simulink model "FOG_v3_1"  (R2023b)
settings: Solver=ode4  StartTime=0.0  StopTime=0.02  FixedStep=2e-08  RelTol=1e-3
undefined symbols (not defined in the file): a_lp, b_lp, eta_conn, eta_dep, eta_K1, eta_pol, f_mod, K1_detector_ratio, K1_launch_ratio, K_norm, K_phase_to_deg, K_ref, K_sag, K_sagnac_power, Omega_deg_s, P_source_W, phi0, Rpd, Rtia, tau, visibility
settings Model: Creator=molik  LastModifiedBy=molik

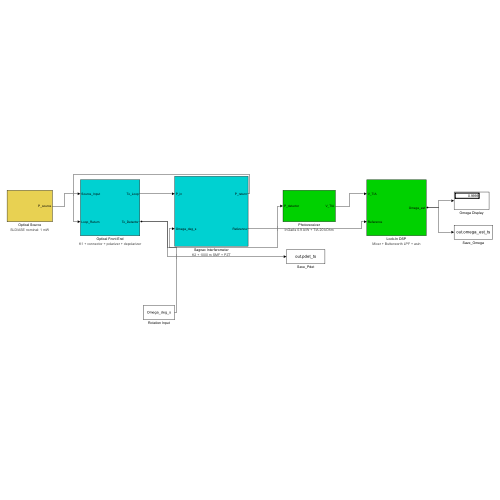
[thumbnail: Simulink's stored preview of the top-level diagram]
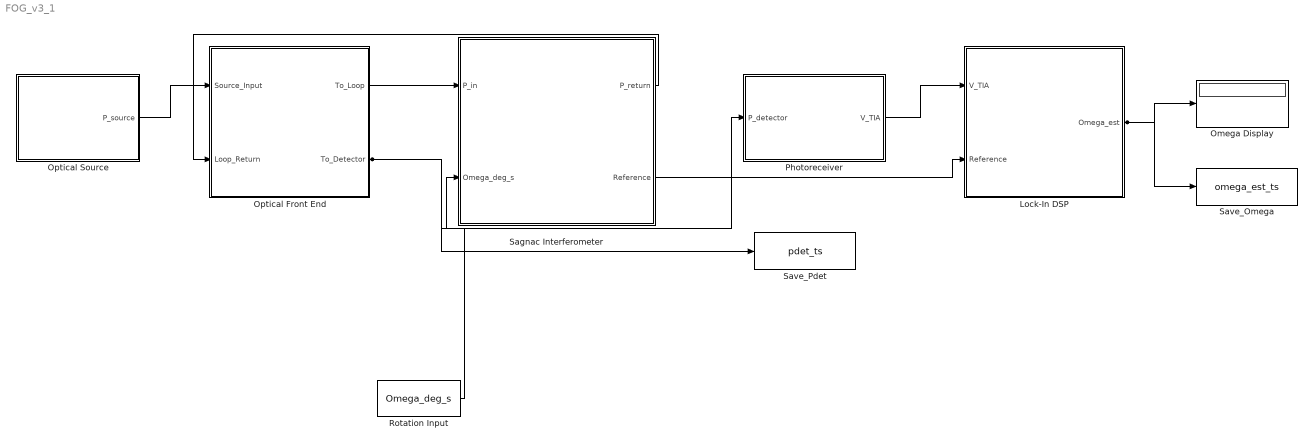
== system FOG_v3_1 ==
  Lock-In DSP : Subsystem
      settings: AttributesFormatString=Mixer + Butterworth LPF + asin
  Omega Display : Display
  Optical Front End : Subsystem
      settings: AttributesFormatString=K1 + connector + polarizer + depolarizer
  Optical Source : Subsystem
      settings: AttributesFormatString=SLD/ASE nominal: 1 mW
  Photoreceiver : Subsystem
      settings: AttributesFormatString=InGaAs 0.9 A/W + TIA 20 kOhm
  Rotation Input : Constant  Value=Omega_deg_s
  Sagnac Interferometer : Subsystem
      settings: AttributesFormatString=K2 + 1000 m SMF + PZT
  Save_Omega : ToWorkspace  VariableName=omega_est_ts  SaveFormat=Timeseries  SampleTime=-1
  Save_Pdet : ToWorkspace  VariableName=pdet_ts  SaveFormat=Timeseries  SampleTime=-1
  wires:
  Optical Source/1(P_source) -> Optical Front End/1(Source_Input)
  Optical Front End/1(To_Loop) -> Sagnac Interferometer/1(P_in)
  Rotation Input/1 -> Sagnac Interferometer/2(Omega_deg_s)
  Sagnac Interferometer/1(P_return) -> Optical Front End/2(Loop_Return)
  Optical Front End/2(To_Detector) -> Photoreceiver/1(P_detector), Save_Pdet/1
  Photoreceiver/1(V_TIA) -> Lock-In DSP/1(V_TIA)
  Sagnac Interferometer/2(Reference) -> Lock-In DSP/2(Reference)
  Lock-In DSP/1(Omega_est) -> Omega Display/1, Save_Omega/1

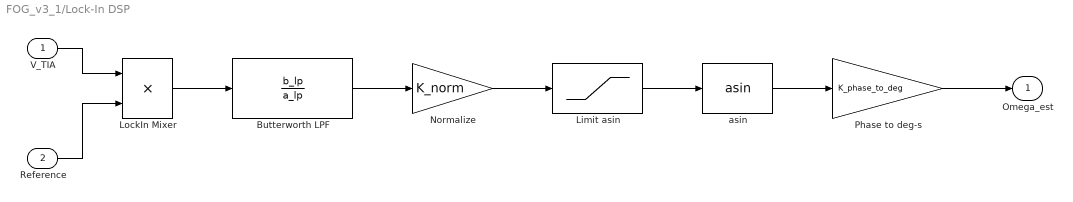
== system FOG_v3_1/Lock-In DSP ==
  V_TIA : Inport
  Reference : Inport  Port=2
  Butterworth LPF : TransferFcn  Numerator=b_lp  Denominator=a_lp
  Limit asin : Saturate  UpperLimit=0.999999  LowerLimit=-0.999999
  LockIn Mixer : Product
  Normalize : Gain  Gain=K_norm
  Phase to deg-s : Gain  Gain=K_phase_to_deg
  asin : Trigonometry  Operator=asin
  Omega_est : Outport
  wires:
  V_TIA/1 -> LockIn Mixer/1
  Reference/1 -> LockIn Mixer/2
  LockIn Mixer/1 -> Butterworth LPF/1
  Butterworth LPF/1 -> Normalize/1
  Normalize/1 -> Limit asin/1
  Limit asin/1 -> asin/1
  asin/1 -> Phase to deg-s/1
  Phase to deg-s/1 -> Omega_est/1

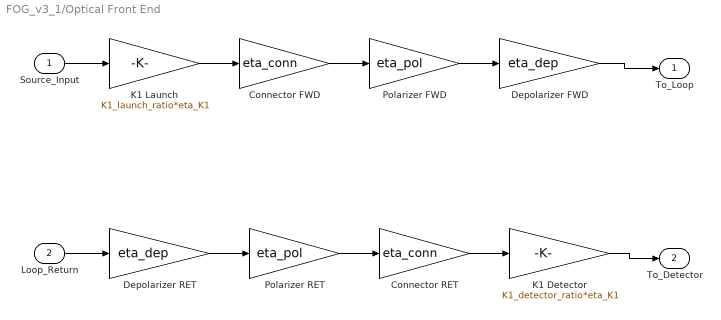
== system FOG_v3_1/Optical Front End ==
  Source_Input : Inport
  Loop_Return : Inport  Port=2
  Connector FWD : Gain  Gain=eta_conn
  Connector RET : Gain  Gain=eta_conn
  Depolarizer FWD : Gain  Gain=eta_dep
  Depolarizer RET : Gain  Gain=eta_dep
  K1 Detector : Gain  Gain=K1_detector_ratio*eta_K1
  K1 Launch : Gain  Gain=K1_launch_ratio*eta_K1
  Polarizer FWD : Gain  Gain=eta_pol
  Polarizer RET : Gain  Gain=eta_pol
  To_Loop : Outport
  To_Detector : Outport  Port=2
  wires:
  Source_Input/1 -> K1 Launch/1
  K1 Launch/1 -> Connector FWD/1
  Connector FWD/1 -> Polarizer FWD/1
  Polarizer FWD/1 -> Depolarizer FWD/1
  Depolarizer FWD/1 -> To_Loop/1
  Loop_Return/1 -> Depolarizer RET/1
  Depolarizer RET/1 -> Polarizer RET/1
  Polarizer RET/1 -> Connector RET/1
  Connector RET/1 -> K1 Detector/1
  K1 Detector/1 -> To_Detector/1

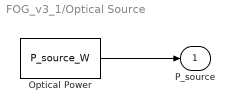
== system FOG_v3_1/Optical Source ==
  Optical Power : Constant  Value=P_source_W
  P_source : Outport
  wires:
  Optical Power/1 -> P_source/1

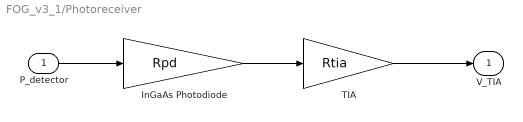
== system FOG_v3_1/Photoreceiver ==
  P_detector : Inport
  InGaAs Photodiode : Gain  Gain=Rpd
  TIA : Gain  Gain=Rtia
  V_TIA : Outport
  wires:
  P_detector/1 -> InGaAs Photodiode/1
  InGaAs Photodiode/1 -> TIA/1
  TIA/1 -> V_TIA/1

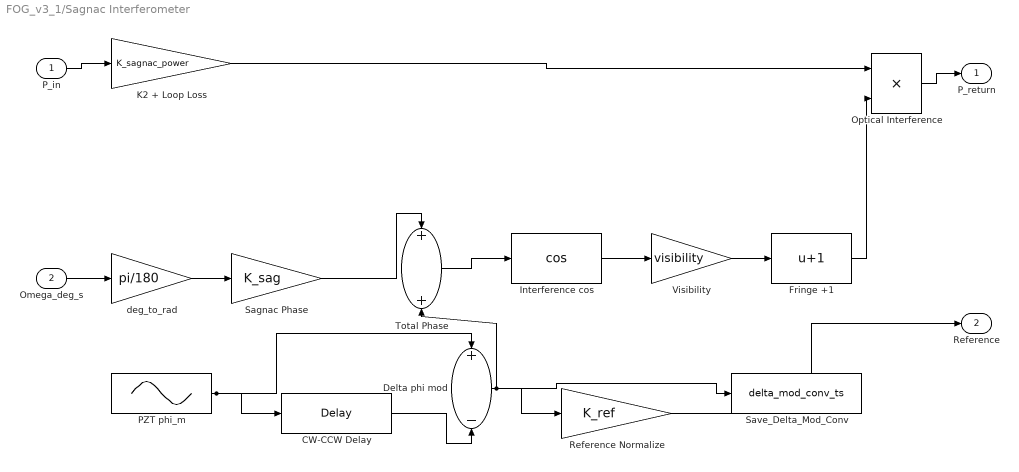
== system FOG_v3_1/Sagnac Interferometer ==
  P_in : Inport
  Omega_deg_s : Inport  Port=2
  CW-CCW Delay : TransportDelay  DelayTime=tau
  Delta phi mod : Sum  Inputs=+-
  Fringe +1 : Bias  Bias=1  SaturateOnIntegerOverflow=off
  Interference cos : Trigonometry  Operator=cos
  K2 + Loop Loss : Gain  Gain=K_sagnac_power
  Optical Interference : Product
  PZT phi_m : Sin  Amplitude=phi0  Frequency=2*pi*f_mod  SampleTime=0
  Reference Normalize : Gain  Gain=K_ref
  Sagnac Phase : Gain  Gain=K_sag
  Save_Delta_Mod_Conv : ToWorkspace  VariableName=delta_mod_conv_ts  SaveFormat=Timeseries  SampleTime=-1
  Total Phase : Sum
  Visibility : Gain  Gain=visibility
  deg_to_rad : Gain  Gain=pi/180
  P_return : Outport
  Reference : Outport  Port=2
  wires:
  P_in/1 -> K2 + Loop Loss/1
  K2 + Loop Loss/1 -> Optical Interference/1
  Omega_deg_s/1 -> deg_to_rad/1
  deg_to_rad/1 -> Sagnac Phase/1
  Sagnac Phase/1 -> Total Phase/1
  PZT phi_m/1 -> Delta phi mod/1, CW-CCW Delay/1
  CW-CCW Delay/1 -> Delta phi mod/2
  Delta phi mod/1 -> Total Phase/2, Reference Normalize/1, Save_Delta_Mod_Conv/1
  Total Phase/1 -> Interference cos/1
  Interference cos/1 -> Visibility/1
  Visibility/1 -> Fringe +1/1
  Fringe +1/1 -> Optical Interference/2
  Optical Interference/1 -> P_return/1
  Reference Normalize/1 -> Reference/1
